simulink model "Hierarcical_controller_temp_"  (R2022b)
settings: Solver=VariableStepAuto  StartTime=0.0  StopTime=120  RelTol=1e-3
InitFcn:
  | %% INITIALIZATION
  | 
  | %% UAV PARAMETERS
  | 
  | mass = 2;
  | Ib = diag([1.2416 1.2416 2*1.2416]);
  | 
  | %% SAMPLING TIME
  | Ts=0.001;
  | 
  | %% PLANNER
  | t_iniz = 0;
  | ttot=20; %duration
  | tdead=10; %dead time to evaluate the steady-state
  | tot_time = ttot + tdead;
  | t1=linspace(0,ttot,round(ttot/Ts));
  | t=linspace(0,ttot+tdead,round(ttot/Ts)+round(tdead/Ts));
  | p= zeros(4,length(t1)); dot_p= zeros(4,length(t1)); ddot_p= zeros(4,length(t1));
  | p_d= zeros(4,length(t)); dot_p_d= zeros(4,length(t)); ddot_p_d= zeros(4,length(t));
  | %Initial and final conditions
  | x0= 0; xf=1; dot_x0= 0; dot_xf=0; ddot_x0=0; ddot_xf=0; dddot_x0 = 0; dddot_xf = 0;
  | y0= 0; yf=1; dot_y0= 0; dot_yf=0; ddot_y0=0; ddot_yf=0; dddot_y0 = 0; dddot_yf = 0;
  | z0= -1; zf=-4; dot_z0= 0; dot_zf=0; ddot_z0=0; ddot_zf=0; dddot_z0 = 0; dddot_zf = 0;
  | psi0 = 0;
  | psif=deg2rad(20); dot_psi0= 0; dot_psif=0; ddot_psi0=0; ddot_psif=0; dddot_psi0 = 0; dddot_psif = 0;
  | p0=[x0,y0,z0,psi0]; dot_p0=[dot_x0,dot_y0,dot_z0,dot_psi0]; ddot_p0=[ddot_x0,ddot_y0,ddot_z0,ddot_psi0]; dddot_p0=[dddot_x0,dddot_y0,dddot_z0,dddot_psi0];
  | pf=[xf,yf,zf,psif]; dot_pf=[dot_xf,dot_yf,dot_zf,dot_psif]; ddot_pf=[ddot_xf,ddot_yf,ddot_zf,ddot_psif]; dddot_pf=[dddot_xf,dddot_yf,dddot_zf,dddot_psif];
  | %5-th order polynomial
  | a0=zeros(1,4); a1=zeros(1,4); a2=zeros(1,4); a3=zeros(1,4); a4=zeros(1,4); a5=zeros(1,4); a6 = zeros(1,4); a7 = zeros(1,4);
  | 
  | for j=1:4
  |     A = [t_iniz^7, t_iniz^6, t_iniz^5, t_iniz^4, t_iniz^3, t_iniz^2, t_iniz, 1;
  |         ttot^7, ttot^6, ttot^5, ttot^4, ttot^3, ttot^2, ttot, 1;
  |         7*t_iniz^6, 6*t_iniz^5, 5*t_iniz^4, 4*t_iniz^3, 3*t_iniz^2, 2*t_iniz, 1, 0;
  |         7*ttot^6, 6*ttot^5, 5*ttot^4, 4*ttot^3, 3*ttot^2, 2*ttot, 1, 0;
  |         42*t_iniz^5, 30*t_iniz^4, 20*t_iniz^3, 12*t_iniz^2, 6*t_iniz, 2, 0, 0;
  |         42*ttot^5, 30*ttot^4, 20*ttot^3, 12*ttot^2, 6*ttot, 2, 0, 0;
  |         210*t_iniz^4, 120*t_iniz^3, 60*t_iniz^2, 24*t_iniz, 6, 0, 0, 0;
  |         210*ttot^4, 120*ttot^3, 60*ttot^2, 24*ttot, 6, 0, 0, 0];
  |     b = [p0(j) pf(j) dot_p0(j) dot_pf(j) ddot_p0(j) ddot_pf(j) dddot_p0(j) dddot_pf(j)]';
  |     a_temp = A\b;
  |     a7(j) = a_temp(1);
  |     a6(j) = a_temp(2);
  |     a5(j) = a_temp(3);
  |     a4(j) = a_temp(4);
  |     a3(j) = a_temp(5);
  |     a2(j) = a_temp(6);
  |     a1(j) = a_temp(7);
  |     a0(j) = a_temp(8);
  | 
  |     %trajectories
  |     p(j,:)=a7(j)*t1.^7 + a6(j)*t1.^6 + a5(j)*t1.^5 +a4(j)*t1.^4 +a3(j)*t1.^3 +a2(j)*t1.^2 +a1(j)*t1 +a0(j);
  |     dot_p(j,:) = 7*a7(j)*t1.^6 + 6*a6(j)*t1.^5 + 5*a5(j)*t1.^4 +4*a4(j)*t1.^3 +3*a3(j)*t1.^2 +2*a2(j)*t1 +a1(j);
  |     ddot_p(j,:) = 42*a7(j)*t1.^5 + 30*a6(j)*t1.^4 + 5*4*a5(j)*t1.^3 +4*3*a4(j)*t1.^2 +3*2*a3(j)*t1 +2*a2(j);
  |     %addition of the stead-state terms
  |     p_d(j,:)=[p(j,:) zeros(1,round(tdead/Ts))+pf(j)];
  |     dot_p_d(j,:)=[dot_p(j,:) zeros(1,round(tdead/Ts))+dot_pf(j)];
  |     ddot_p_d(j,:)=[ddot_p(j,:) zeros(1,round(tdead/Ts))+ddot_pf(j)];
  | end
  | %data for Simulink
  | pos_0 = [x0 y0 z0];
  | lin_vel_0 = [dot_x0 dot_y0 dot_z0];
  | w_bb_0 = [0 0 0];
  | eta_b_0 = [0 0 0];
  | eta_b_dot_0 = [0 0 0];
values from neighbouring files (symbols this model uses):
  Track_path = DFS(A_adj,2,path)    [BRRT_3D.m]    (also in GOOD_PATH.mat = [3 15.8545082605 15.9232549014 27.6290043449 38.9996108348 4)
libraries: robotcorelib x1, uavutilslib x1
settings Model: Creator=fabioruggiero  LastModifiedBy=storm
settings ModelReferenceCC: EnableRefExpFcnMdlSchedulingChecks=on

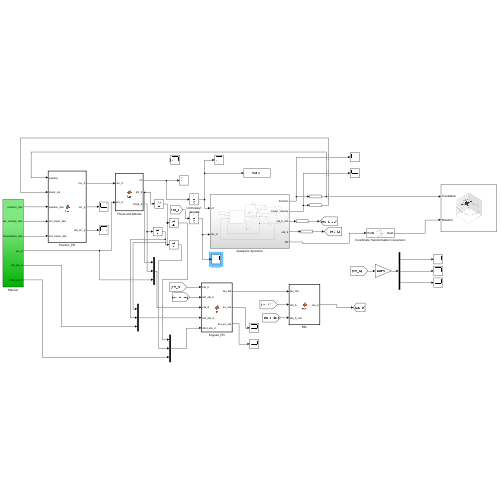
[thumbnail: Simulink's stored preview of the top-level diagram]
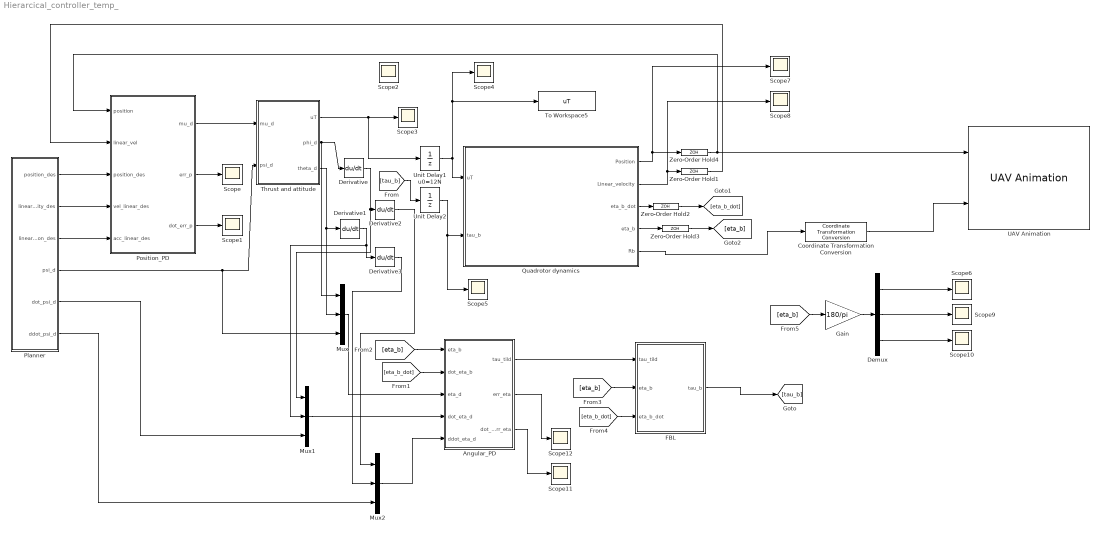
== system Hierarcical_controller_temp_ ==
  Angular_PD : MATLAB Function  TreatAsAtomicUnit=on
  Coordinate Transformation Conversion : robotcorelib/Coordinate Transformation Conversion  InputRepresentation=Rotation Matrix  InputEulerSequence=ZYX  ShowTrVecInputPort=on  OutputRepresentation=Quaternion  OutputEulerSequence=XYZ  ShowTrVecOutputPort=on  SimulateUsing=Interpreted execution
  Demux : Demux  Outputs=3
  Derivative{,1..3} (4 alike) : Derivative
  FBL : MATLAB Function  TreatAsAtomicUnit=on
  Gain : Gain  Gain=180/pi
  Mux : Mux  Inputs=3
  Mux1 : Mux  Inputs=3
  Mux2 : Mux  Inputs=3
  Planner : Subsystem
  Position_PD : MATLAB Function  TreatAsAtomicUnit=on
  Quadrotor dynamics : Subsystem
  Scope{,1..12} (13 alike) : Scope
  Thrust and attitude : MATLAB Function  TreatAsAtomicUnit=on
  To Workspace5 : ToWorkspace  VariableName=uT  SaveFormat=Structure With Time  SampleTime=-1
  UAV Animation : uavutilslib/UAV Animation  UAVType=Multirotor  UAVSize=1  InertialZDirection=Down  SampleTime=0.01
  Unit Delay1 u0=12N : UnitDelay  InitialCondition=mass*9.81  SampleTime=Ts
  Unit Delay2 : UnitDelay  InitialCondition=[0 0 0]  SampleTime=Ts
  Zero-Order Hold{1..4} (4 alike) : ZeroOrderHold  SampleTime=Ts
  wires:
  Planner/2(linear_velocity_des) -> Position_PD/4(vel_linear_des)
  Unit Delay2/1 -> Quadrotor dynamics/2(tau_b), Scope5/1
  Planner/1(position_des) -> Position_PD/3(position_des)
  Quadrotor dynamics/2(Linear_velocity) -> Scope8/1, Zero-Order Hold1/1
  Quadrotor dynamics/1(Position) -> Scope7/1, Zero-Order Hold4/1
  Coordinate Transformation Conversion/1 -> UAV Animation/2
  Position_PD/3(dot_err_p) -> Scope1/1
  Position_PD/2(err_p) -> Scope/1
  Planner/3(linear_acceleration_des) -> Position_PD/5(acc_linear_des)
  Unit Delay1 u0=12N/1 -> Quadrotor dynamics/1(uT), Scope4/1, To Workspace5/1
  Zero-Order Hold1/1 -> Position_PD/2(linear_vel)
  Position_PD/1(mu_d) -> Thrust and attitude/1(mu_d)
  Thrust and attitude/1(uT) -> Unit Delay1 u0=12N/1, Scope3/1
  Planner/4(psi_d) -> Mux/3, Thrust and attitude/2(psi_d)
  Thrust and attitude/2(phi_d) -> Mux/1, Derivative/1
  Thrust and attitude/3(theta_d) -> Mux/2, Derivative1/1
  Derivative/1 -> Mux1/1, Derivative2/1
  Derivative1/1 -> Mux1/2, Derivative3/1
  Mux/1 -> Angular_PD/3(eta_d)
  Planner/5(dot_psi_d) -> Mux1/3
  Mux1/1 -> Angular_PD/4(dot_eta_d)
  Derivative2/1 -> Mux2/1
  Derivative3/1 -> Mux2/2
  Planner/6(ddot_psi_d) -> Mux2/3
  Mux2/1 -> Angular_PD/5(ddot_eta_d)
  Angular_PD/1(tau_tild) -> FBL/1(tau_tild)
  FBL/1(tau_b) -> [tau_b]
  [tau_b] -> Unit Delay2/1
  Quadrotor dynamics/3(eta_b_dot) -> Zero-Order Hold2/1
  Quadrotor dynamics/4(eta_b) -> Zero-Order Hold3/1
  Zero-Order Hold2/1 -> [eta_b_dot]
  [eta_b_dot] -> Angular_PD/2(dot_eta_b)
  Zero-Order Hold3/1 -> [eta_b]
  [eta_b] -> Angular_PD/1(eta_b)
  [eta_b] -> FBL/2(eta_b)
  [eta_b_dot] -> FBL/3(eta_b_dot)
  [eta_b] -> Gain/1
  Demux/1 -> Scope6/1
  Demux/2 -> Scope9/1
  Demux/3 -> Scope10/1
  Gain/1 -> Demux/1
  Angular_PD/2(err_eta) -> Scope12/1
  Angular_PD/3(dot_err_eta) -> Scope11/1
  Zero-Order Hold4/1 -> UAV Animation/1, Position_PD/1(position)
  Quadrotor dynamics/5(Rb) -> Coordinate Transformation Conversion/1

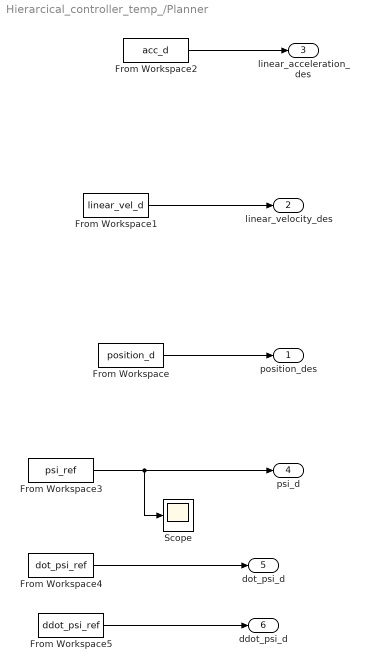
== system Hierarcical_controller_temp_/Planner ==
  From Workspace : FromWorkspace  VariableName=position_d
  From Workspace1 : FromWorkspace  VariableName=linear_vel_d
  From Workspace2 : FromWorkspace  VariableName=acc_d
  From Workspace3 : FromWorkspace  VariableName=psi_ref
  From Workspace4 : FromWorkspace  VariableName=dot_psi_ref
  From Workspace5 : FromWorkspace  VariableName=ddot_psi_ref
  Scope : Scope
  position_des : Outport
  linear_velocity_des : Outport  Port=2
  linear_acceleration_des : Outport  Port=3
  psi_d : Outport  Port=4
  dot_psi_d : Outport  Port=5
  ddot_psi_d : Outport  Port=6
  wires:
  From Workspace/1 -> position_des/1
  From Workspace1/1 -> linear_velocity_des/1
  From Workspace2/1 -> linear_acceleration_des/1
  From Workspace3/1 -> Scope/1, psi_d/1
  From Workspace4/1 -> dot_psi_d/1
  From Workspace5/1 -> ddot_psi_d/1

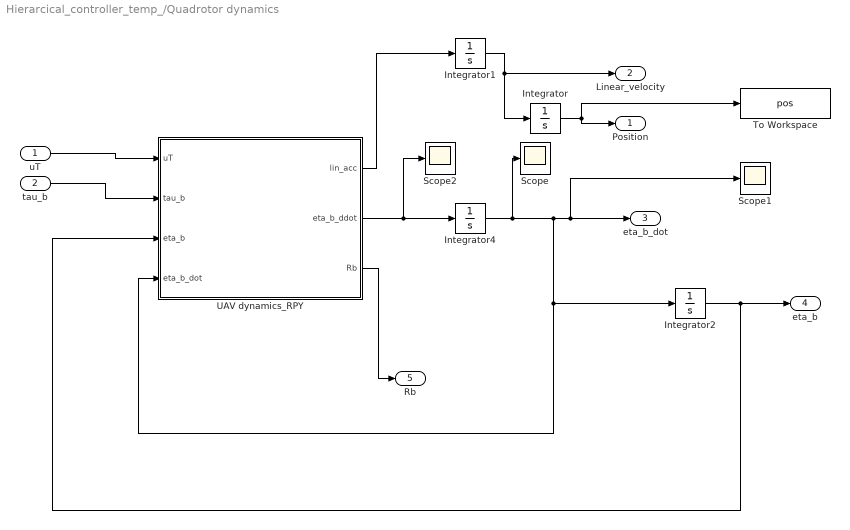
== system Hierarcical_controller_temp_/Quadrotor dynamics ==
  uT : Inport
  tau_b : Inport  Port=2
  Integrator : Integrator  InitialCondition=Track_path(1,:)
  Integrator1 : Integrator  InitialCondition=lin_vel_0
  Integrator2 : Integrator  InitialCondition=eta_b_0
  Integrator4 : Integrator  InitialCondition=eta_b_dot_0
  Scope : Scope
  Scope1 : Scope
  Scope2 : Scope
  To Workspace : ToWorkspace  VariableName=pos  SaveFormat=Structure With Time  SampleTime=-1
  UAV dynamics_RPY : MATLAB Function  TreatAsAtomicUnit=on
  Position : Outport
  Linear_velocity : Outport  Port=2
  eta_b_dot : Outport  Port=3
  eta_b : Outport  Port=4
  Rb : Outport  Port=5
  wires:
  tau_b/1 -> UAV dynamics_RPY/2(tau_b)
  UAV dynamics_RPY/1(lin_acc) -> Integrator1/1
  uT/1 -> UAV dynamics_RPY/1(uT)
  Integrator1/1 -> Integrator/1, Linear_velocity/1
  Integrator/1 -> Position/1, To Workspace/1
  Integrator4/1 -> Scope/1, UAV dynamics_RPY/4(eta_b_dot), Integrator2/1, Scope1/1, eta_b_dot/1
  Integrator2/1 -> UAV dynamics_RPY/3(eta_b), eta_b/1
  UAV dynamics_RPY/3(Rb) -> Rb/1
  UAV dynamics_RPY/2(eta_b_ddot) -> Integrator4/1, Scope2/1

== matlab function Hierarcical_controller_temp_/Position_PD ==
  data: position input; mu_d output; linear_vel input; position_des input; vel_linear_des input; acc_linear_des input; err_p output; dot_err_p output
function [mu_d, err_p, dot_err_p] = fcn(position, linear_vel,position_des, vel_linear_des, acc_linear_des)

Kp=[5*eye(3) 5*eye(3)];
err_p=position-position_des;
dot_err_p=linear_vel-vel_linear_des;

mu_d=-Kp*[err_p;dot_err_p]+acc_linear_des;

end

== matlab function Hierarcical_controller_temp_/Thrust and attitude ==
  data: mu_d input; uT output; psi_d input; phi_d output; theta_d output; mass parameter size=1
function [uT, phi_d, theta_d] = fcn(mu_d,psi_d,mass)

g=9.81;

uT=mass*sqrt(mu_d(1)^2+mu_d(2)^2+(mu_d(3)-g)^2);

phi_d=asin((mass/uT)*(mu_d(2)*cos(psi_d)-mu_d(1)*sin(psi_d)));

theta_d=atan((mu_d(1)*cos(psi_d)+mu_d(2)*sin(psi_d))/(mu_d(3)-g));

end

== matlab function Hierarcical_controller_temp_/Angular_PD ==
  data: eta_b input; tau_tild output; dot_eta_b input; eta_d input; dot_eta_d input; ddot_eta_d input; err_eta output; dot_err_eta output
function [tau_tild ,err_eta, dot_err_eta] = fcn(eta_b,dot_eta_b,eta_d,dot_eta_d,ddot_eta_d)

Ke=[30*eye(3) 30*eye(3)];
err_eta=eta_b-eta_d;
dot_err_eta=dot_eta_b-dot_eta_d;

tau_tild=-Ke*[err_eta;dot_err_eta]+ddot_eta_d;




end

== matlab function Hierarcical_controller_temp_/FBL ==
  data: tau_tild input; tau_b output size=3; eta_b input; eta_b_dot input; Ib parameter
function tau_b = fcn(tau_tild,eta_b,eta_b_dot,Ib)


Q=Q_fun(eta_b);
C=C_fun(eta_b,eta_b_dot,Ib);


tau_b= Ib*Q*tau_tild + inv(Q)'*C*eta_b_dot;
end


function S=skew(w)

if(numel(w)~= 1)

S= [0 -w(3) w(2);
w(3) 0 -w(1);
-w(2) w(1) 0];

else

S= zeros(3);

end

end



function Q = Q_fun(RPY)
Q=[1 0 -sin(RPY(2));
    0 cos(RPY(1)) cos(RPY(2))*sin(RPY(1))
    0 -sin(RPY(1)) cos(RPY(1))*cos(RPY(2))];
end

function Q_dot=Q_dot_fun(eta_b,eta_b_dot)

 
Q_dot=[0 0 -cos(eta_b(2))*eta_b_dot(2);

0 -sin(eta_b(1))*eta_b_dot(1) -sin(eta_b(2))*sin(eta_b(1))*eta_b_dot(2)+cos(eta_b(2))*cos(eta_b(1))*eta_b_dot(1);

0 -cos(eta_b(1))*eta_b_dot(1) -sin(eta_b(2))*cos(eta_b(1))*eta_b_dot(2)-cos(eta_b(2))*sin(eta_b(1))*eta_b_dot(1)];

end





function C=C_fun(eta_b,eta_b_dot,Ib)
Q=Q_fun(eta_b);
S=skew(Q*eta_b_dot);
Q_dot=Q_dot_fun(eta_b,eta_b_dot);
C=Q'*S*Ib*Q+Q'*Ib*Q_dot;
end

== matlab function Hierarcical_controller_temp_/Quadrotor dynamics/UAV dynamics_RPY ==
  data: uT input size=1; tau_b input size=3; lin_acc output size=3; eta_b input size=3; eta_b_dot input; mass parameter size=1; Ib parameter size=[3,3]; eta_b_ddot output size=3; Rb output
function [lin_acc,eta_b_ddot,Rb] = fcn(uT,tau_b,eta_b,eta_b_dot,mass, Ib)

M=M_fun(eta_b,Ib);
C=C_fun(eta_b,eta_b_dot,Ib);
Q=Q_fun(eta_b);
Rb=R_fun(eta_b);

lin_acc = 9.81*[0 0 1]'-(uT/mass)*Rb*[0 0 1]';


eta_b_ddot=inv(M)*(-C*eta_b_dot+Q'*tau_b);


end

function S=skew(w)

if(numel(w)~= 1)

S= [0 -w(3) w(2);
w(3) 0 -w(1);
-w(2) w(1) 0];

else

S= zeros(3);

end

end

function Q_dot=Q_dot_fun(eta_b,eta_b_dot)

 
Q_dot=[0 0 -cos(eta_b(2))*eta_b_dot(2);

0 -sin(eta_b(1))*eta_b_dot(1) -sin(eta_b(2))*sin(eta_b(1))*eta_b_dot(2)+cos(eta_b(2))*cos(eta_b(1))*eta_b_dot(1);

0 -cos(eta_b(1))*eta_b_dot(1) -sin(eta_b(2))*cos(eta_b(1))*eta_b_dot(2)-cos(eta_b(2))*sin(eta_b(1))*eta_b_dot(1)];

end



function M=M_fun(eta_b,Ib)

Q=Q_fun(eta_b);

M=Q'*Ib*Q;


end


function C=C_fun(eta_b,eta_b_dot,Ib)

Q=Q_fun(eta_b);
S=skew(Q*eta_b_dot);
Q_dot=Q_dot_fun(eta_b,eta_b_dot);
C=Q'*S*Ib*Q+Q'*Ib*Q_dot;


end

function Q = Q_fun(RPY)
Q=[1 0 -sin(RPY(2));
    0 cos(RPY(1)) cos(RPY(2))*sin(RPY(1))
    0 -sin(RPY(1)) cos(RPY(1))*cos(RPY(2))];
end

function Rb = R_fun(eta_b)
Rb=[cos(eta_b(2))*cos(eta_b(3)) sin(eta_b(1))*sin(eta_b(2))*cos(eta_b(3))-cos(eta_b(1))*sin(eta_b(3)) cos(eta_b(1))*sin(eta_b(2))*cos(eta_b(3))+sin(eta_b(1))*sin(eta_b(3));
    cos(eta_b(2))*sin(eta_b(3)) sin(eta_b(1))*sin(eta_b(2))*sin(eta_b(3))+cos(eta_b(1))*cos(eta_b(3)) cos(eta_b(1))*sin(eta_b(2))*sin(eta_b(3))-sin(eta_b(1))*cos(eta_b(3));
-sin(eta_b(2)) sin(eta_b(1))*cos(eta_b(2)) cos(eta_b(1))*cos(eta_b(2))];
end
